simulink model "example_Absorption_Chiller_LookUp"  (R2016b)
settings: Solver=ode45  StartTime=0.0  StopTime=5000  FixedStep=1  MaxStep=120  RelTol=1e-3  EnableMultiTasking=on
PreLoadFcn:
  | % load Yazaki_KF.mat;
libraries: carnot x9, simulink_extras x6, simulink x4
settings Model: Creator=Simulation  LastModifiedBy=awohlfei
settings DataIOCC: LimitDataPoints=on  SaveFormat=Array  SignalLoggingSaveFormat=ModelDataLogs
settings OptimizationCC: ExpressionDepthLimit=2147483647  LifeSpan=inf
settings DebuggingCC: SolverPrmCheckMsg=warning  StateNameClashWarn=warning  SFUnexpectedBacktrackingDiag=warning  SFNoUnconditionalDefaultTransitionDiag=warning  SFExecutionAtInitializationDiag=none
settings HardwareCC: ProdBitPerPointer=32  ProdBitPerSizeT=32  ProdBitPerPtrDiffT=32  ProdLargestAtomicFloat=None  ProdIntDivRoundTo=Undefined  ProdEndianess=Unspecified  ProdWordSize=32  ProdHWDeviceType=32-bit Generic
settings ModelReferenceCC: PropagateSignalLabelsOutOfModel=off
settings GRTTargetCC: TargetLangStandard=C89/C90 (ANSI)  GeneratePreprocessorConditionals=Disable all  CombineOutputUpdateFcns=off  GRTInterface=on
settings ConfigComp: CovMetricSettings=dw  CovHtmlReporting=on  CovSaveCumulativeToWorkspaceVar=on  CovSaveSingleToWorkspaceVar=on  CovExternalEMLEnable=off

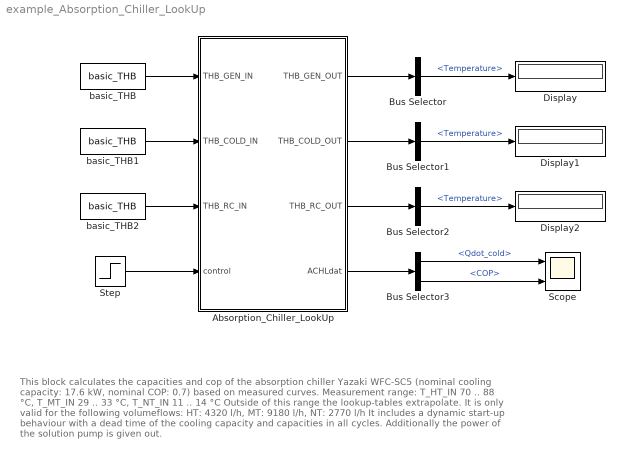
== system example_Absorption_Chiller_LookUp ==
  note: This block calculates the capacities and cop of the absorption chiller Yazaki WFC-SC5 (nominal cooling capacity: 17.6 kW, nominal COP: 0.7) based on measured curves.
      | Measurement range:
      | T_HT_IN 70 .. 88 °C, T_MT_IN 29 .. 33 °C, T_NT_IN 11 .. 14 °C
      | Outside of this range the lookup-tables extrapolate.
      |
      | It is only valid for the following volumeflows:
      | HT: 4320 l/h, MT: 9180 l/h, NT: 2770 l/h
      |
      | It includes a dynamic start-up behaviour with a dead time of the cooling capacity and capacities in all cycles.
      | Additionally the power of the solution pump is given out.
  Absorption_Chiller_LookUp : Subsystem  AncestorBlock=carnot/Source/Chiller/Absorption_Chiller_LookUp  LoadFcn=|  mask(Absorption_Chiller_LookUp){chillertype=Yazaki WFC-SC5, heating_T_heating=[70 71 72 73 74 75 76 77 78 79 80 81 82 83 84 85 86 87 88], heating_T_recooling=[29 31 33], heating_T_cooling=[11 12.5 14], heating_Qdot=1000*cat(3, [11.5881 9.1729 7.1257; 12.7010 10.3602 8.4661; 13.7629 11.4453 9.5786; 14.7846 12.4541 10.5382; 15.7779 13.4104 11.3994; 16.7568 14.3365 12.1994; 17.7369 15.2538 12.9661; 18.7352 16.1871 13.7316; 19.7725 17.1783 14.5620; 20.8727 18.2790 15.5386; 21.4613 18.7997 16.0051; 22.1221 19.4526 16.6571; 22.8301 20.1885 17.4171; 23.5620 20.9610 18.2116; 24.3132 21.7625 19.0310; 25.0838 22.5963 19.8849; 25.8734 23.4650 20.7822; 26.6798 24.3672 21.7227; 27.5000 25.3000 22.7026], [11.5770 9.1404 7.0019; 12.7946 10.4820 8.5464; 13.9519 11.6809 9.7954; 15.0589 12.7736 10.8503; 16.1256 13.7910 11.7810; 17.1622 14.7571 12.6313; 18.1791 15.6924 13.4319; 19.1897 16.6217 14.2164; 20.2208 17.5967 15.0560; 21.3053 18.6810 16.0354; 21.9686 19.2406 16.5703; 22.7017 19.9403 17.2856; 23.4728 20.7187 18.0972; 24.2533 21.5195 18.9268; 25.0400 22.3359 19.7666; 25.8372 23.1759 20.6298; 26.6482 24.0459 21.5289; 27.4705 24.9436 22.4620; 28.3000 25.8635 23.4225], [11.6060 9.2707 7.0732; 12.8444 10.5919 8.6463; 14.0314 11.8008 9.9499; 15.1740 12.9258 11.0711; 16.2788 13.9911 12.0715; 17.3504 15.0094 12.9866; 18.3927 15.9884 13.8393; 19.4114 16.9403 14.6560; 20.4215 17.9043 15.5008; 21.4421 18.9298 16.4494; 22.3770 19.7105 17.1376; 23.3307 20.5777 17.9644; 24.2859 21.4864 18.8566; 25.2275 22.3953 19.7465; 26.1572 23.3020 20.6298; 27.0823 24.2153 21.5215; 28.0081 25.1426 22.4350; 28.9326 26.0813 23.3675; 29.8510 27.0252 24.3106]), recooling_T_heating=[70 79 88], recooling_T_recooling=[29 31 33], recooling_T_cooling=[11 12.5 14], recooling_Qdot=1000*cat(3, [17.7490 12.9282 8.7004; 34.7262 30.2580 25.0504; 45.9087 40.8416 35.7528], [17.2271 12.0716 8.2439; 35.4258 31.2730 26.0419; 48.6320 43.2955 38.4385], [17.2978 12.4414 8.1943; 35.0711 30.8160 26.3417; 52.3435 45.8810 40.5337]), cooling_T_heating=[70 79 88], cooling_T_recooling=[29 31 33], cooling_T_cooling=[11 12.5 14], cooling_Qdot=1000*cat(3, [7.0144 4.7740 2.6867; 14.9294 12.8469 10.4033; 19.0103 16.2646 13.7101], [6.8604 4.4520 2.5150; 15.2614 13.2863 10.9945; 20.4077 17.6879 15.3832], [6.9061 4.7080 2.6441; 15.1135 13.2179 11.1459; 22.6100 19.5272 17.0154]), deadtime_factor=11768, deadtime_exponent=-1.205}
      | load('THB.mat');
      | CarnotCallbacks_Absorption_Chiller_LookUp('CreateMaskStyles', gcb);
      | CarnotCallbacks_Absorption_Chiller_LookUp('CreateMaskVisibilities', gcb);
      mask prompts: chillertype "chiller type"; heating_T_heating "T heating beakpoints"; heating_T_recooling "T recooling beakpoints"; heating_T_cooling "T cooling beakpoints"; heating_Qdot "Q generator table"; recooling_T_heating "T heating beakpoints"; recooling_T_recooling "T recooling beakpoints"; recooling_T_cooling "T cooling beakpoints"; recooling_Qdot "Q recooling table"; cooling_T_heating "T heating beakpoints"; cooling_T_recooling "T recooling beakpoints"; cooling_T_cooling "T cooling beakpoints"; cooling_Qdot "Q cooling table"; deadtime_factor "factor"; deadtime_exponent "exponent"
      mask help: This block calculates the capacities and cop of an absorption chiller via a lookup table.
      mask init:
      | data = CarnotCallbacks_Absorption_Chiller_LookUp('GetChillerData', chillertype, heating_T_heating, heating_T_recooling, heating_T_cooling, heating_Qdot, recooling_T_heating, recooling_T_recooling, recooling_T_cooling, recooling_Qdot, cooling_T_heating, cooling_T_recooling, cooling_T_cooling, cooling_Qdot, deadtime_factor, deadtime_exponent);
      settings: AttributesFormatString=%<chillertype>
      mask Help: eval('helpcarnot')
      mask TypeOptions chillertype: Yazaki WFC-SC5 | own data
      mask Callback chillertype: CarnotCallbacks_Absorption_Chiller_LookUp('CreateMaskVisibilities', gcb);
  Bus Selector : BusSelector  OutputSignals=Temperature
  Bus Selector1 : BusSelector  OutputSignals=Temperature
  Bus Selector2 : BusSelector  OutputSignals=Temperature
  Bus Selector3 : BusSelector  OutputSignals=Qdot_cold,COP
  Display : Display
  Display1 : Display
  Display2 : Display
  Scope : Scope  NumInputPorts=2
  Step : Step  Time=600  SampleTime=0
  basic_THB : carnot/Basic/Hydraulics/basic_THB  t=88  mdot=4320/3600  p=1e5  ID=Pressure Drop from Massflow  fluid=Water  mix=0  mix2=0  mix3=0  dia=0.02  hgt=0
  basic_THB1 : carnot/Basic/Hydraulics/basic_THB  t=12.5  mdot=2770/3600  p=1e5  ID=Pressure Drop from Massflow  fluid=Water  mix=0  mix2=0  mix3=0  dia=0.02  hgt=0
  basic_THB2 : carnot/Basic/Hydraulics/basic_THB  t=31  mdot=9180/3600  p=1e5  ID=Pressure Drop from Massflow  fluid=Water  mix=0  mix2=0  mix3=0  dia=0.02  hgt=0
  wires:
  basic_THB/1 -> Absorption_Chiller_LookUp/1(THB_GEN_IN)
  basic_THB1/1 -> Absorption_Chiller_LookUp/2(THB_COLD_IN)
  basic_THB2/1 -> Absorption_Chiller_LookUp/3(THB_RC_IN)
  Step/1 -> Absorption_Chiller_LookUp/4(control)
  Absorption_Chiller_LookUp/1(THB_GEN_OUT) -> Bus Selector/1
  Bus Selector/1 -> Display/1  "<Temperature>"
  Absorption_Chiller_LookUp/2(THB_COLD_OUT) -> Bus Selector1/1
  Bus Selector1/1 -> Display1/1  "<Temperature>"
  Bus Selector2/1 -> Display2/1  "<Temperature>"
  Absorption_Chiller_LookUp/3(THB_RC_OUT) -> Bus Selector2/1
  Absorption_Chiller_LookUp/4(ACHLdat) -> Bus Selector3/1
  Bus Selector3/1 -> Scope/1  "<Qdot_cold>"
  Bus Selector3/2 -> Scope/2  "<COP>"

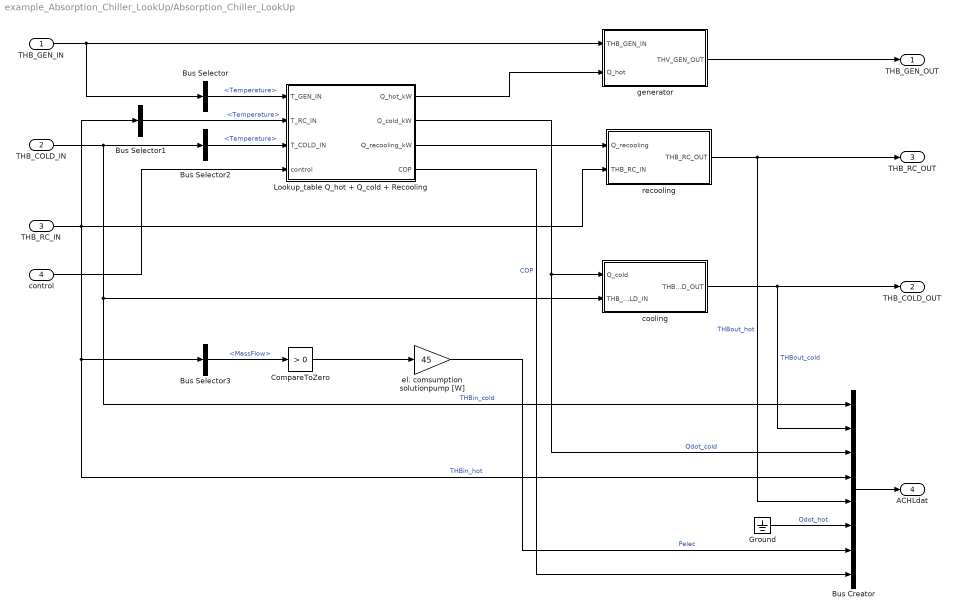
== system example_Absorption_Chiller_LookUp/Absorption_Chiller_LookUp ==
  THB_GEN_IN : Inport  OutDataTypeStr=Bus: THB
  THB_COLD_IN : Inport  Port=2  OutDataTypeStr=Bus: THB
  THB_RC_IN : Inport  Port=3  OutDataTypeStr=Bus: THB
  control : Inport  Port=4
  Bus Creator : BusCreator  Inputs=8
  Bus Selector : BusSelector  OutputSignals=Temperature
  Bus Selector1 : BusSelector  OutputSignals=Temperature
  Bus Selector2 : BusSelector  OutputSignals=Temperature
  Bus Selector3 : BusSelector  OutputSignals=MassFlow
  CompareToZero : simulink/Logic and Bit Operations/Compare To Zero  relop=>  OutDataTypeStr=uint8
  Ground : Ground
  Lookup_table Q_hot + Q_cold + Recooling : Subsystem  TreatAsAtomicUnit=on
  cooling : Subsystem
  el. comsumption solutionpump [W] : Gain  Gain=45
  generator : Subsystem
  recooling : Subsystem
  THB_GEN_OUT : Outport
  THB_COLD_OUT : Outport  Port=2
  THB_RC_OUT : Outport  Port=3
  ACHLdat : Outport  Port=4
  wires:
  THB_GEN_IN/1 -> generator/1(THB_GEN_IN), Bus Selector/1
  generator/1(THV_GEN_OUT) -> THB_GEN_OUT/1
  Bus Selector1/1 -> Lookup_table Q_hot + Q_cold + Recooling/2(T_RC_IN)  "<Temperature>"
  control/1 -> Lookup_table Q_hot + Q_cold + Recooling/4(control)
  Bus Selector2/1 -> Lookup_table Q_hot + Q_cold + Recooling/3(T_COLD_IN)  "<Temperature>"
  Lookup_table Q_hot + Q_cold + Recooling/1(Q_hot_kW) -> generator/2(Q_hot)
  Lookup_table Q_hot + Q_cold + Recooling/3(Q_recooling_kW) -> recooling/1(Q_recooling)
  CompareToZero/1 -> el. comsumption solutionpump [W]/1
  Bus Selector/1 -> Lookup_table Q_hot + Q_cold + Recooling/1(T_GEN_IN)  "<Temperature>"
  Lookup_table Q_hot + Q_cold + Recooling/4(COP) -> Bus Creator/8  "COP"
  Bus Selector3/1 -> CompareToZero/1  "<MassFlow>"
  Bus Creator/1 -> ACHLdat/1
  cooling/1(THB_COLD_OUT) -> Bus Creator/2, THB_COLD_OUT/1  "THBout_cold"
  THB_COLD_IN/1 -> Bus Creator/1, cooling/2(THB_COLD_IN), Bus Selector2/1  "THBin_cold"
  recooling/1(THB_RC_OUT) -> THB_RC_OUT/1, Bus Creator/5  "THBout_hot"
  THB_RC_IN/1 -> Bus Creator/4, Bus Selector3/1, Bus Selector1/1, recooling/2(THB_RC_IN)  "THBin_hot"
  el. comsumption solutionpump [W]/1 -> Bus Creator/7  "Pelec"
  Lookup_table Q_hot + Q_cold + Recooling/2(Q_cold_kW) -> cooling/1(Q_cold), Bus Creator/3  "Qdot_cold"
  Ground/1 -> Bus Creator/6  "Qdot_hot"

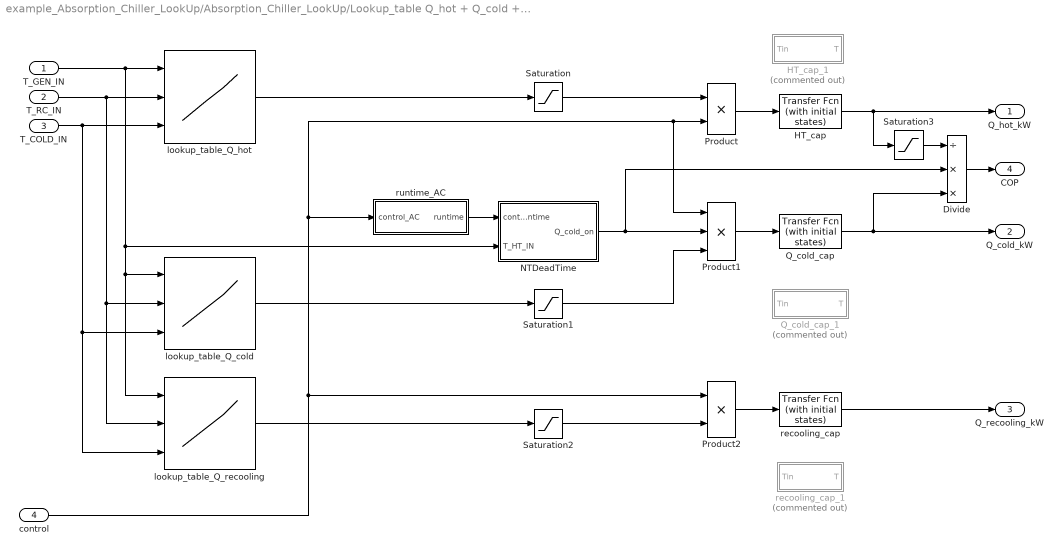
== system example_Absorption_Chiller_LookUp/Absorption_Chiller_LookUp/Lookup_table Q_hot + Q_cold + Recooling ==
  T_GEN_IN : Inport
  T_RC_IN : Inport  Port=2
  T_COLD_IN : Inport  Port=3
  control : Inport  Port=4
  Divide : Product  Inputs=/**
  HT_cap : simulink_extras/Additional Linear/Transfer Fcn (with initial states)  N=[1]  D="[21.55  1]"  X0=0
  HT_cap_1 : Subsystem  Commented=on  mask(capacity){NTU=0.0464, Tini=0}
      mask prompts: NTU "heat transfer / heat capacity NTU (k*A/(m*cp))"; Tini "initial temperature [degree centigrade]"
      mask help: The block introduces a capacity of the component. It can be used to break an algebraic loop.
      mask Help: eval('man(''capacity'')')
  NTDeadTime : Subsystem
  Product : Product  RndMeth=Zero
  Product1 : Product  Inputs=3  RndMeth=Zero
  Product2 : Product  RndMeth=Zero
  Q_cold_cap : simulink_extras/Additional Linear/Transfer Fcn (with initial states)  N=[1]  D="[52.356  1]"  X0=0
  Q_cold_cap_1 : Subsystem  Commented=on  mask(capacity){NTU=0.0191, Tini=0}
      mask prompts: NTU "heat transfer / heat capacity NTU (k*A/(m*cp))"; Tini "initial temperature [degree centigrade]"
      mask help: The block introduces a capacity of the component. It can be used to break an algebraic loop.
      mask Help: eval('man(''capacity'')')
  Saturation : Saturate  UpperLimit=inf  LowerLimit=0
  Saturation1 : Saturate  UpperLimit=inf  LowerLimit=0
  Saturation2 : Saturate  UpperLimit=inf  LowerLimit=0
  Saturation3 : Saturate  UpperLimit=inf  LowerLimit=eps(10)  ZeroCross=off
  lookup_table_Q_cold : Lookup_n-D  NumberOfTableDimensions=3  BreakpointsForDimension1=data.cooling_T_heating  BreakpointsForDimension2=data.cooling_T_recooling  BreakpointsForDimension3=data.cooling_T_cooling  BreakpointsForDimension4=[1:2]  Table=data.cooling_Qdot  InputSameDT=on
  lookup_table_Q_hot : Lookup_n-D  NumberOfTableDimensions=3  BreakpointsForDimension1=data.heating_T_heating  BreakpointsForDimension2=data.heating_T_recooling  BreakpointsForDimension3=data.heating_T_cooling  BreakpointsForDimension4=[1:2]  Table=data.heating_Qdot  InputSameDT=on
  lookup_table_Q_recooling : Lookup_n-D  NumberOfTableDimensions=3  BreakpointsForDimension1=data.recooling_T_heating  BreakpointsForDimension2=data.recooling_T_recooling  BreakpointsForDimension3=data.recooling_T_cooling  BreakpointsForDimension4=[1:2]  Table=data.recooling_Qdot  InputSameDT=on
  recooling_cap : simulink_extras/Additional Linear/Transfer Fcn (with initial states)  N=[1]  D="[104.17  1]"  X0=0
  recooling_cap_1 : Subsystem  Commented=on  mask(capacity){NTU=0.0096, Tini=0}
      mask prompts: NTU "heat transfer / heat capacity NTU (k*A/(m*cp))"; Tini "initial temperature [degree centigrade]"
      mask help: The block introduces a capacity of the component. It can be used to break an algebraic loop.
      mask Help: eval('man(''capacity'')')
  runtime_AC : Subsystem  TreatAsAtomicUnit=on
      mask help: This block counts the time if input is set to one, it stops counting if input is zero and continues when input rises to one again.
      mask Help: eval('filetest (''manual.htm#count_working_time'')')
  Q_hot_kW : Outport
  Q_cold_kW : Outport  Port=2
  Q_recooling_kW : Outport  Port=3
  COP : Outport  Port=4
  wires:
  T_COLD_IN/1 -> lookup_table_Q_cold/3, lookup_table_Q_recooling/3, lookup_table_Q_hot/3
  T_RC_IN/1 -> lookup_table_Q_cold/2, lookup_table_Q_recooling/2, lookup_table_Q_hot/2
  T_GEN_IN/1 -> lookup_table_Q_cold/1, lookup_table_Q_recooling/1, NTDeadTime/2(T_HT_IN), lookup_table_Q_hot/1
  lookup_table_Q_hot/1 -> Saturation/1
  control/1 -> Product/2, Product1/1, runtime_AC/1(control_AC), Product2/1
  runtime_AC/1(runtime) -> NTDeadTime/1(control_AC_runtime)
  Product/1 -> HT_cap/1
  Product1/1 -> Q_cold_cap/1
  HT_cap/1 -> Q_hot_kW/1, Saturation3/1
  Q_cold_cap/1 -> Q_cold_kW/1, Divide/3
  lookup_table_Q_cold/1 -> Saturation1/1
  recooling_cap/1 -> Q_recooling_kW/1
  Product2/1 -> recooling_cap/1
  lookup_table_Q_recooling/1 -> Saturation2/1
  Saturation/1 -> Product/1
  Saturation1/1 -> Product1/3
  Saturation2/1 -> Product2/2
  Divide/1 -> COP/1
  NTDeadTime/1(Q_cold_on) -> Divide/2, Product1/2
  Saturation3/1 -> Divide/1

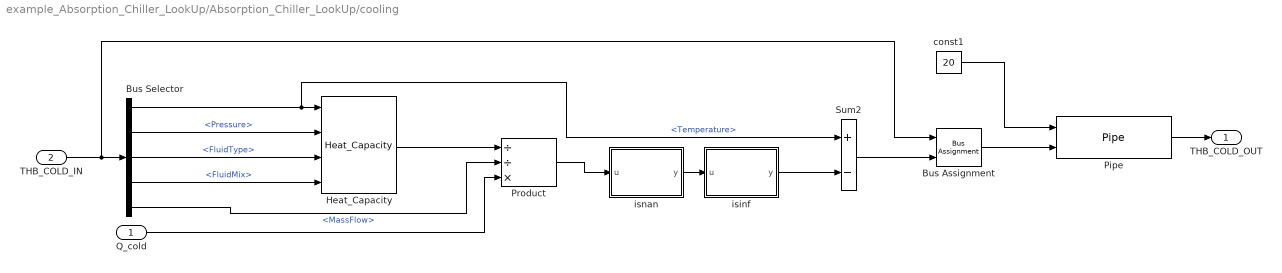
== system example_Absorption_Chiller_LookUp/Absorption_Chiller_LookUp/cooling ==
  Q_cold : Inport
  THB_COLD_IN : Inport  Port=2  OutDataTypeStr=Bus: THB
  Bus Assignment : BusAssignment  AssignedSignals=Temperature
  Bus Selector : BusSelector  OutputSignals=Temperature,Pressure,FluidType,FluidMix,MassFlow
  Heat_Capacity : carnot/Basic/Material_Properties/Heat_Capacity  VariantControl=CarlibClassic  INPUTARGUMENTS=state variables (classic)  DEBUGLEVEL=DEBUGLEVEL  MAXTOTALWARNINGS=inf  MAXCONSECUTIVEWARNINGS=inf  WRITETOFILE=0  FILENAME='errors.txt'
  Pipe : carnot/Hydraulics/Pipe  dia=0.02  len=10  hgt=5  uloss=100/20/10  cond=0  cwall=1000  t0=20  lin=100/0.2  qua=100/0.2^2  nodes=10
  Product : Product  Inputs=//*  SaturateOnIntegerOverflow=on  RndMeth=Zero  InputSameDT=on  OutDataTypeStr=Inherit: Same as first input
  Sum2 : Sum  Inputs=+-  InputSameDT=on  OutDataTypeStr=Inherit: Same as first input
  const1 : Constant  Value=20
  isinf : MATLAB Function  TreatAsAtomicUnit=on
  isnan : MATLAB Function  TreatAsAtomicUnit=on
  THB_COLD_OUT : Outport
  wires:
  Heat_Capacity/1 -> Product/1
  THB_COLD_IN/1 -> Bus Assignment/1, Bus Selector/1
  Bus Selector/1 -> Sum2/1, Heat_Capacity/1  "<Temperature>"
  Bus Selector/2 -> Heat_Capacity/2  "<Pressure>"
  Bus Selector/3 -> Heat_Capacity/3  "<FluidType>"
  Bus Selector/4 -> Heat_Capacity/4  "<FluidMix>"
  isnan/1(y) -> isinf/1(u)
  Product/1 -> isnan/1(u)
  isinf/1(y) -> Sum2/2
  Bus Selector/5 -> Product/2  "<MassFlow>"
  Sum2/1 -> Bus Assignment/2
  Pipe/1 -> THB_COLD_OUT/1
  Bus Assignment/1 -> Pipe/2
  const1/1 -> Pipe/1
  Q_cold/1 -> Product/3

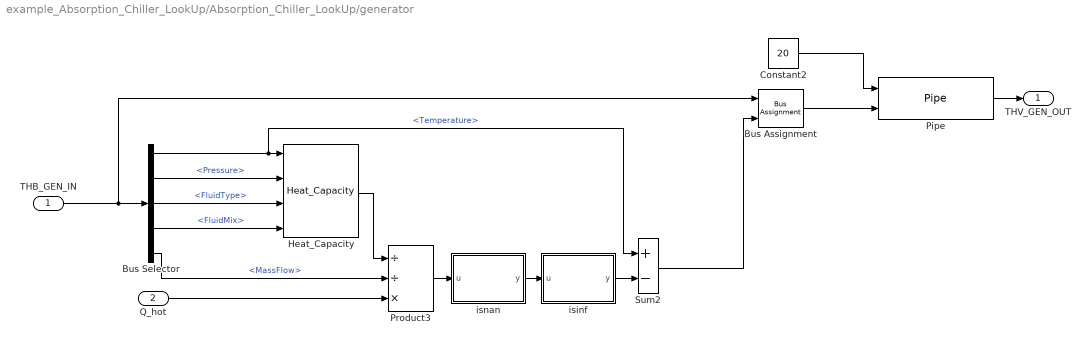
== system example_Absorption_Chiller_LookUp/Absorption_Chiller_LookUp/generator ==
  THB_GEN_IN : Inport
  Q_hot : Inport  Port=2
  Bus Assignment : BusAssignment  AssignedSignals=Temperature
  Bus Selector : BusSelector  OutputSignals=Temperature,Pressure,FluidType,FluidMix,MassFlow
  Constant2 : Constant  Value=20
  Heat_Capacity : carnot/Basic/Material_Properties/Heat_Capacity  VariantControl=CarlibClassic  INPUTARGUMENTS=state variables (classic)  DEBUGLEVEL=DEBUGLEVEL  MAXTOTALWARNINGS=inf  MAXCONSECUTIVEWARNINGS=inf  WRITETOFILE=0  FILENAME='errors.txt'
  Pipe : carnot/Hydraulics/Pipe  dia=0.02  len=10  hgt=5  uloss=100/20/10  cond=0  cwall=1000  t0=20  lin=100/0.2  qua=100/0.2^2  nodes=10
  Product3 : Product  Inputs=//*  SaturateOnIntegerOverflow=on  RndMeth=Zero  InputSameDT=on  OutDataTypeStr=Inherit: Same as first input
  Sum2 : Sum  Inputs=+-  InputSameDT=on  OutDataTypeStr=Inherit: Same as first input
  isinf : MATLAB Function  TreatAsAtomicUnit=on
  isnan : MATLAB Function  TreatAsAtomicUnit=on
  THV_GEN_OUT : Outport
  wires:
  Product3/1 -> isnan/1(u)
  Heat_Capacity/1 -> Product3/1
  Bus Selector/1 -> Sum2/1, Heat_Capacity/1  "<Temperature>"
  Q_hot/1 -> Product3/3
  isnan/1(y) -> isinf/1(u)
  isinf/1(y) -> Sum2/2
  Sum2/1 -> Bus Assignment/2
  Pipe/1 -> THV_GEN_OUT/1
  Constant2/1 -> Pipe/1
  THB_GEN_IN/1 -> Bus Assignment/1, Bus Selector/1
  Bus Selector/2 -> Heat_Capacity/2  "<Pressure>"
  Bus Selector/3 -> Heat_Capacity/3  "<FluidType>"
  Bus Selector/4 -> Heat_Capacity/4  "<FluidMix>"
  Bus Selector/5 -> Product3/2  "<MassFlow>"
  Bus Assignment/1 -> Pipe/2

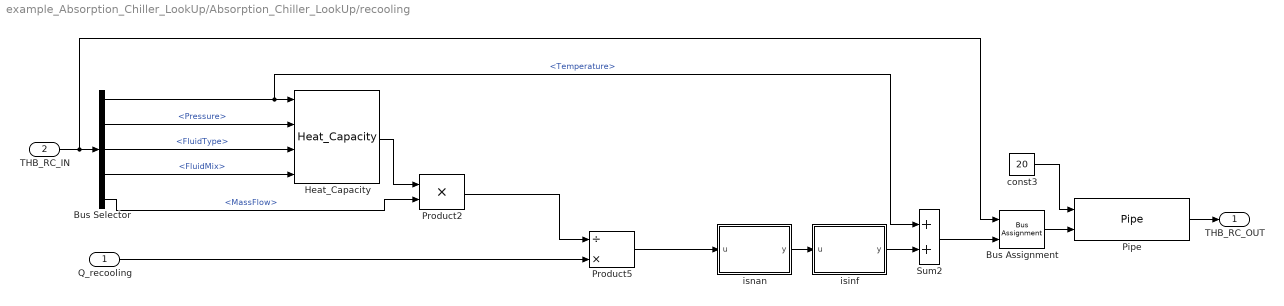
== system example_Absorption_Chiller_LookUp/Absorption_Chiller_LookUp/recooling ==
  Q_recooling : Inport
  THB_RC_IN : Inport  Port=2
  Bus Assignment : BusAssignment  AssignedSignals=Temperature
  Bus Selector : BusSelector  OutputSignals=Temperature,Pressure,FluidType,FluidMix,MassFlow
  Heat_Capacity : carnot/Basic/Material_Properties/Heat_Capacity  VariantControl=CarlibClassic  INPUTARGUMENTS=state variables (classic)  DEBUGLEVEL=DEBUGLEVEL  MAXTOTALWARNINGS=inf  MAXCONSECUTIVEWARNINGS=inf  WRITETOFILE=0  FILENAME='errors.txt'
  Pipe : carnot/Hydraulics/Pipe  dia=0.02  len=10  hgt=5  uloss=100/20/10  cond=0  cwall=1000  t0=20  lin=100/0.2  qua=100/0.2^2  nodes=10
  Product2 : Product  Inputs=**  SaturateOnIntegerOverflow=on  RndMeth=Zero  InputSameDT=on  OutDataTypeStr=Inherit: Same as first input
  Product5 : Product  Inputs=/*  SaturateOnIntegerOverflow=on  RndMeth=Zero  InputSameDT=on  OutDataTypeStr=Inherit: Same as first input
  Sum2 : Sum  InputSameDT=on  OutDataTypeStr=Inherit: Same as first input
  const3 : Constant  Value=20
  isinf : MATLAB Function  TreatAsAtomicUnit=on
  isnan : MATLAB Function  TreatAsAtomicUnit=on
  THB_RC_OUT : Outport
  wires:
  Q_recooling/1 -> Product5/2
  Product2/1 -> Product5/1
  Bus Selector/5 -> Product2/2  "<MassFlow>"
  Heat_Capacity/1 -> Product2/1
  Bus Selector/2 -> Heat_Capacity/2  "<Pressure>"
  Bus Selector/4 -> Heat_Capacity/4  "<FluidMix>"
  Bus Selector/3 -> Heat_Capacity/3  "<FluidType>"
  Bus Selector/1 -> Sum2/1, Heat_Capacity/1  "<Temperature>"
  isnan/1(y) -> isinf/1(u)
  isinf/1(y) -> Sum2/2
  Sum2/1 -> Bus Assignment/2
  Product5/1 -> isnan/1(u)
  Bus Assignment/1 -> Pipe/2
  Pipe/1 -> THB_RC_OUT/1
  const3/1 -> Pipe/1
  THB_RC_IN/1 -> Bus Assignment/1, Bus Selector/1

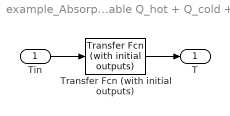
== system example_Absorption_Chiller_LookUp/Absorption_Chiller_LookUp/Lookup_table Q_hot + Q_cold + Recooling/HT_cap_1 ==
  Tin : Inport
  Transfer Fcn (with initial outputs) : simulink_extras/Additional Linear/Transfer Fcn (with initial outputs)  N=[1]  D="[1/NTU  1]"  Y0=Tini  U0=0
  T : Outport
  wires:
  Tin/1 -> Transfer Fcn (with initial outputs)/1
  Transfer Fcn (with initial outputs)/1 -> T/1

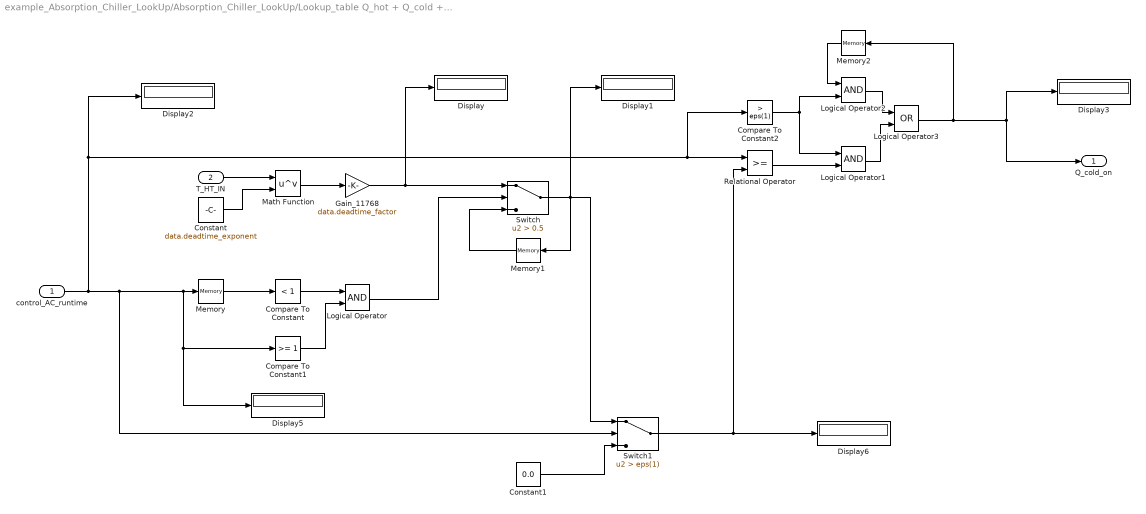
== system example_Absorption_Chiller_LookUp/Absorption_Chiller_LookUp/Lookup_table Q_hot + Q_cold + Recooling/NTDeadTime ==
  control_AC_runtime : Inport
  T_HT_IN : Inport  Port=2
  Compare To Constant : simulink/Logic and Bit Operations/Compare To Constant  relop=<  const=1  OutDataTypeStr=boolean
  Compare To Constant1 : simulink/Logic and Bit Operations/Compare To Constant  relop=>=  const=1  OutDataTypeStr=boolean
  Compare To Constant2 : simulink/Logic and Bit Operations/Compare To Constant  relop=>  const=eps(1)  OutDataTypeStr=boolean
  Constant : Constant  Value=data.deadtime_exponent
  Constant1 : Constant  Value=0.0
  Display{,1..3,5..6} (6 alike) : Display
  Gain_11768 : Gain  Gain=data.deadtime_factor
  Logical Operator : Logic  AllPortsSameDT=off  OutDataTypeStr=boolean
  Logical Operator1 : Logic  AllPortsSameDT=off  OutDataTypeStr=boolean
  Logical Operator2 : Logic  AllPortsSameDT=off  OutDataTypeStr=boolean
  Logical Operator3 : Logic  Operator=OR  AllPortsSameDT=off  OutDataTypeStr=boolean
  Math Function : Math  Operator=pow  SaturateOnIntegerOverflow=on
  Memory : Memory
  Memory1 : Memory
  Memory2 : Memory
  Relational Operator : RelationalOperator  OutDataTypeStr=boolean  RndMeth=Simplest
  Switch : Switch  Criteria=u2 > Threshold  Threshold=0.5
  Switch1 : Switch  Criteria=u2 > Threshold  Threshold=eps(1)
  Q_cold_on : Outport
  wires:
  T_HT_IN/1 -> Math Function/1
  Constant/1 -> Math Function/2
  Math Function/1 -> Gain_11768/1
  Gain_11768/1 -> Display/1, Switch/1
  Memory/1 -> Compare To Constant/1
  Compare To Constant/1 -> Logical Operator/1
  Logical Operator/1 -> Switch/2
  Switch/1 -> Switch1/1, Memory1/1, Display1/1
  Memory1/1 -> Switch/3
  control_AC_runtime/1 -> Display2/1, Compare To Constant2/1, Relational Operator/1, Switch1/2, Display5/1, Compare To Constant1/1, Memory/1
  Constant1/1 -> Switch1/3
  Compare To Constant1/1 -> Logical Operator/2
  Switch1/1 -> Display6/1, Relational Operator/2
  Relational Operator/1 -> Logical Operator1/2
  Compare To Constant2/1 -> Logical Operator1/1, Logical Operator2/2
  Memory2/1 -> Logical Operator2/1
  Logical Operator2/1 -> Logical Operator3/1
  Logical Operator3/1 -> Memory2/1, Display3/1, Q_cold_on/1
  Logical Operator1/1 -> Logical Operator3/2

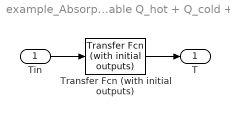
== system example_Absorption_Chiller_LookUp/Absorption_Chiller_LookUp/Lookup_table Q_hot + Q_cold + Recooling/Q_cold_cap_1 ==
  Tin : Inport
  Transfer Fcn (with initial outputs) : simulink_extras/Additional Linear/Transfer Fcn (with initial outputs)  N=[1]  D="[1/NTU  1]"  Y0=Tini  U0=0
  T : Outport
  wires:
  Tin/1 -> Transfer Fcn (with initial outputs)/1
  Transfer Fcn (with initial outputs)/1 -> T/1

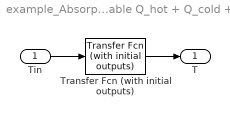
== system example_Absorption_Chiller_LookUp/Absorption_Chiller_LookUp/Lookup_table Q_hot + Q_cold + Recooling/recooling_cap_1 ==
  Tin : Inport
  Transfer Fcn (with initial outputs) : simulink_extras/Additional Linear/Transfer Fcn (with initial outputs)  N=[1]  D="[1/NTU  1]"  Y0=Tini  U0=0
  T : Outport
  wires:
  Tin/1 -> Transfer Fcn (with initial outputs)/1
  Transfer Fcn (with initial outputs)/1 -> T/1

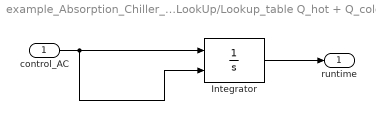
== system example_Absorption_Chiller_LookUp/Absorption_Chiller_LookUp/Lookup_table Q_hot + Q_cold + Recooling/runtime_AC ==
  control_AC : Inport
  Integrator : Integrator  ExternalReset=either
  runtime : Outport
  wires:
  control_AC/1 -> Integrator/2, Integrator/1
  Integrator/1 -> runtime/1

== matlab function example_Absorption_Chiller_LookUp/Absorption_Chiller_LookUp/cooling/isinf ==
  data: u input; y output

function y = fcn(u)

%Verhindert die Fehlerausgabe bei Teilen mit dem Wert 0 
%Dieser Zustand tritt ein wenn der Volumenstrom 0 l/s gesetzt wird.

v = isinf (u);

if v == 0
    
    y = u;

else 
    
    y = 0;
    
end

== matlab function example_Absorption_Chiller_LookUp/Absorption_Chiller_LookUp/cooling/isnan ==
  data: u input; y output

function y = fcn(u)

%Verhindert die Fehlerausgabe bei Teilen durch den Wert 0 
%Dieser Zustand tritt ein wenn der Volumenstrom 0 l/s gesetzt wird.

v = isnan (u);

if v == 0
    
    y = u;

else 
    
    y = 0;
    
end

== matlab function example_Absorption_Chiller_LookUp/Absorption_Chiller_LookUp/generator/isinf ==
  data: u input; y output

function y = fcn(u)

%Verhindert die Fehlerausgabe bei Teilen mit dem Wert 0 
%Dieser Zustand tritt ein wenn der Volumenstrom 0 l/s gesetzt wird.

v = isinf (u);

if v == 0
    
    y = u;

else 
    
    y = 0;
    
end

== matlab function example_Absorption_Chiller_LookUp/Absorption_Chiller_LookUp/generator/isnan ==
  data: u input; y output

function y = fcn(u)

%Verhindert die Fehlerausgabe bei Teilen durch den Wert 0 
%Dieser Zustand tritt ein wenn der Volumenstrom 0 l/s gesetzt wird.

v = isnan (u);

if v == 0
    
    y = u;

else 
    
    y = 0;
    
end

== matlab function example_Absorption_Chiller_LookUp/Absorption_Chiller_LookUp/recooling/isinf ==
  data: u input; y output

function y = fcn(u)

%Verhindert die Fehlerausgabe bei Teilen mit dem Wert 0 
%Dieser Zustand tritt ein wenn der Volumenstrom 0 l/s gesetzt wird.

v = isinf (u);

if v == 0
    
    y = u;

else 
    
    y = 0;
    
end

== matlab function example_Absorption_Chiller_LookUp/Absorption_Chiller_LookUp/recooling/isnan ==
  data: u input; y output

function y = fcn(u)

%Verhindert die Fehlerausgabe bei Teilen durch den Wert 0 
%Dieser Zustand tritt ein wenn der Volumenstrom 0 l/s gesetzt wird.

v = isnan (u);

if v == 0
    
    y = u;

else 
    
    y = 0;
    
end
